simulink model "Rocket_Simulink"  (R2024b)
settings: Solver=VariableStepAuto  StartTime=0.0  StopTime=50  RelTol=1e-3
values from neighbouring files (symbols this model uses):
  A_alt = [ ... (first row only)    [linear_model.m]
  A_att = [ ... (first row only)    [linear_model.m]
  B_alt = [ ... (first row only)    [linear_model.m]
  B_att = [ ... (first row only)    [linear_model.m]
  C_alt = eye(2)    [linear_model.m]
  g = 9.82    [linear_model.m]
  h = 0.4    [linear_model.m]
  K_alt = lqr(A_alt, B_alt, Q_alt, R_alt)    [linear_model.m]
  K_att = K_aug(:, 1:6)    [linear_model.m]
  K_I = K_aug(:, 7)    [linear_model.m]
  m = 3    [linear_model.m]
undefined symbols (not defined in the file or in its folder): C_I
libraries: simulink x3, simulink_extras x1
settings Model: Creator=akewi  LastModifiedBy=akewi

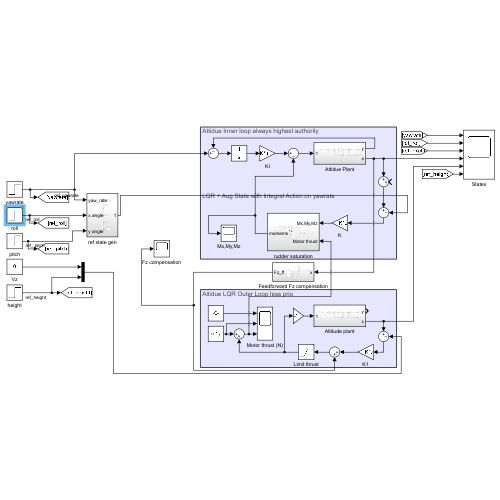
[thumbnail: Simulink's stored preview of the top-level diagram]
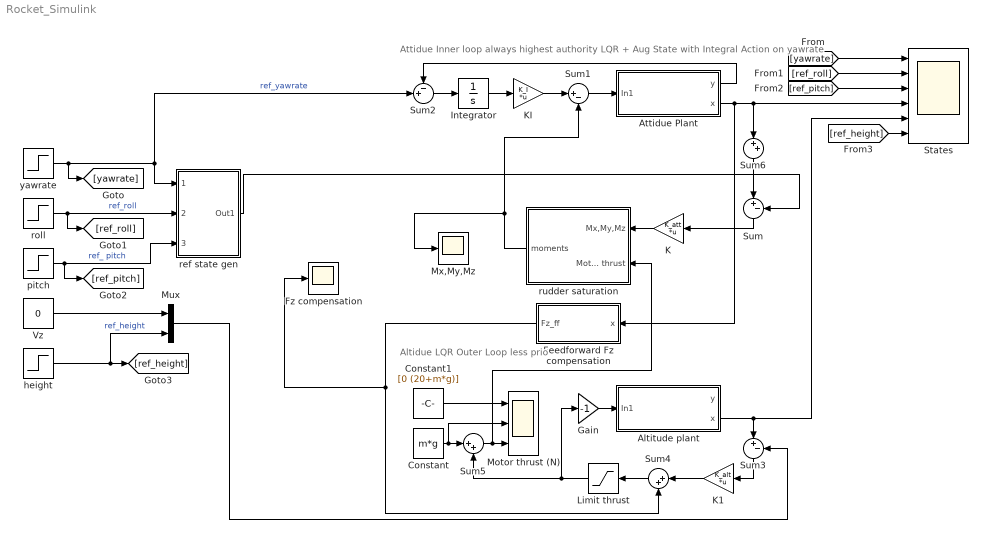
== system Rocket_Simulink ==
  note: Attidue Inner loop always highest authority
      |
      |
      |
      |
      |
      |
      |
      |
      | LQR + Aug State with Integral Action on yawrate
  note: Altidue LQR Outer Loop less prio
  Altitude plant : Subsystem
  Attidue Plant : Subsystem
  Constant : Constant  Value=m*g
  Constant1 : Constant  Value=[0 (20+m*g)]
  Feedforward Fz compensation : Subsystem
  Fz compensation : Scope
  Gain : Gain  Gain=-1
  Integrator : Integrator
  K : Gain  Gain=K_att  Multiplication=Matrix(K*u)
  K1 : Gain  Gain=K_alt  Multiplication=Matrix(K*u)
  KI : Gain  Gain=K_I  Multiplication=Matrix(K*u)
  Limit thrust : Saturate  UpperLimit=20  LowerLimit=-m*g
  Motor thrust (N) : Scope  NumInputPorts=3
  Mux : Mux  Inputs=2
  Mx,My,Mz : Scope
  States : Scope  NumInputPorts=6
  Sum : Sum  Inputs=|+-
  Sum1 : Sum  Inputs=|+-
  Sum2 : Sum  Inputs=-+|
  Sum3 : Sum  Inputs=|+-
  Sum4 : Sum  Inputs=|++
  Sum5 : Sum  Inputs=|++
  Sum6 : Sum  Inputs=|++
  Vz : Constant  Value=0
  height : Step  After=0  SampleTime=0
  pitch : Step  After=0  SampleTime=0
  ref state gen : Subsystem
  roll : Step  Time=3  After=5  SampleTime=0
  rudder saturation : Subsystem
  yawrate : Step  Time=5  After=0  SampleTime=0
  wires:
  yawrate/1 -> [yawrate], ref state gen/1(yaw_rate), Sum2/2  "ref_yawrate"
  roll/1 -> [ref_roll], ref state gen/2(x angle)  "ref_roll"
  pitch/1 -> [ref_pitch], ref state gen/3(y angle)  "ref_ pitch"
  Attidue Plant/2(x) -> Feedforward Fz compensation/1(x), States/4, Sum6/1
  ref state gen/1(Out1) -> Sum/2
  Sum/1 -> K/1
  Attidue Plant/1(y) -> Sum2/1
  Sum1/1 -> Attidue Plant/1(In1)
  KI/1 -> Sum1/1
  Integrator/1 -> KI/1
  Sum2/1 -> Integrator/1
  [yawrate] -> States/1
  [ref_roll] -> States/2
  [ref_pitch] -> States/3
  Limit thrust/1 -> Gain/1, Sum5/2
  Altitude plant/2(x) -> States/5, Sum3/1
  Sum3/1 -> K1/1
  Mux/1 -> Sum3/2
  Vz/1 -> Mux/1
  height/1 -> Mux/2, [ref_height]  "ref_height"
  Sum5/1 -> rudder saturation/2(Motor thrust), Motor thrust (N)/3
  Constant/1 -> Motor thrust (N)/2, Sum5/1
  Constant1/1 -> Motor thrust (N)/1
  Gain/1 -> Altitude plant/1(In1)
  [ref_height] -> States/6
  Sum4/1 -> Limit thrust/1
  K1/1 -> Sum4/1
  Feedforward Fz compensation/1(Fz_ff) -> Fz compensation/1, Sum4/2
  K/1 -> rudder saturation/1(Mx,My,Mz)
  rudder saturation/1(moments) -> Mx,My,Mz/1, Sum1/2
  Sum6/1 -> Sum/1

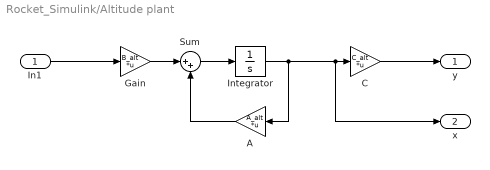
== system Rocket_Simulink/Altitude plant ==
  In1 : Inport
  A : Gain  Gain=A_alt  Multiplication=Matrix(K*u)
  C : Gain  Gain=C_alt  Multiplication=Matrix(K*u)
  Gain : Gain  Gain=B_alt  Multiplication=Matrix(K*u)
  Integrator : Integrator
  Sum : Sum  Inputs=|++
  y : Outport
  x : Outport  Port=2
  wires:
  Integrator/1 -> A/1, x/1, C/1
  C/1 -> y/1
  A/1 -> Sum/2
  Sum/1 -> Integrator/1
  Gain/1 -> Sum/1
  In1/1 -> Gain/1

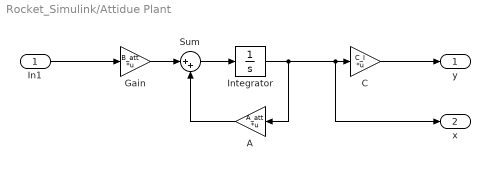
== system Rocket_Simulink/Attidue Plant ==
  In1 : Inport
  A : Gain  Gain=A_att  Multiplication=Matrix(K*u)
  C : Gain  Gain=C_I  Multiplication=Matrix(K*u)
  Gain : Gain  Gain=B_att  Multiplication=Matrix(K*u)
  Integrator : Integrator
  Sum : Sum  Inputs=|++
  y : Outport
  x : Outport  Port=2
  wires:
  Integrator/1 -> A/1, x/1, C/1
  C/1 -> y/1
  A/1 -> Sum/2
  Sum/1 -> Integrator/1
  Gain/1 -> Sum/1
  In1/1 -> Gain/1

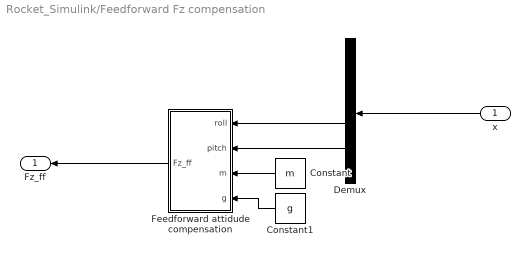
== system Rocket_Simulink/Feedforward Fz compensation ==
  x : Inport
  Constant : Constant  Value=m
  Constant1 : Constant  Value=g
  Demux : Demux  Outputs=6
  Feedforward attidude compensation : MATLAB Function  TreatAsAtomicUnit=on
  Fz_ff : Outport
  wires:
  x/1 -> Demux/1
  Feedforward attidude compensation/1(Fz_ff) -> Fz_ff/1
  Demux/4 -> Feedforward attidude compensation/1(roll)
  Demux/5 -> Feedforward attidude compensation/2(pitch)
  Constant/1 -> Feedforward attidude compensation/3(m)
  Constant1/1 -> Feedforward attidude compensation/4(g)

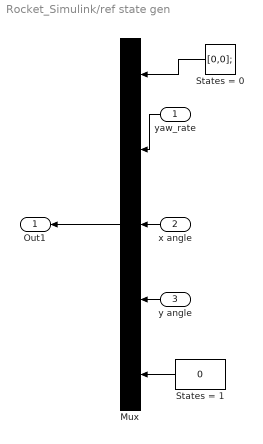
== system Rocket_Simulink/ref state gen ==
  yaw_rate : Inport
  x angle : Inport  Port=2
  y angle : Inport  Port=3
  Mux : Mux  Inputs=5
  States = 0 : Constant  Value=[0,0];
  States = 1 : Constant  Value=0
  Out1 : Outport
  wires:
  x angle/1 -> Mux/3
  States = 1/1 -> Mux/5
  y angle/1 -> Mux/4
  States = 0/1 -> Mux/1
  yaw_rate/1 -> Mux/2
  Mux/1 -> Out1/1

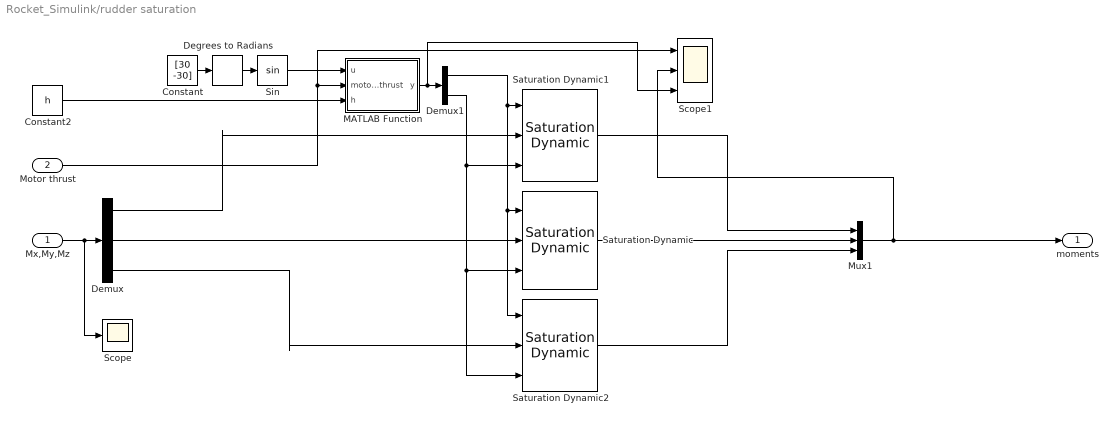
== system Rocket_Simulink/rudder saturation ==
  Mx,My,Mz : Inport
  Motor thrust : Inport  Port=2
  Constant : Constant  Value=[30 -30]
  Constant2 : Constant  Value=h
  Degrees to Radians : simulink_extras/Transformations/Degrees to Radians
  Demux : Demux  Outputs=3
  Demux1 : Demux  Outputs=2
  MATLAB Function : MATLAB Function  TreatAsAtomicUnit=on
  Mux1 : Mux  Inputs=3
  Saturation Dynamic : simulink/Discontinuities/Saturation Dynamic  OutMin=[]  OutMax=[]  OutDataTypeStr=Inherit: Same as second input  OutDataType=fixdt(1, 16)  OutScaling=2^-10  DoSatur=off
  Saturation Dynamic1 : simulink/Discontinuities/Saturation Dynamic  OutMin=[]  OutMax=[]  OutDataTypeStr=Inherit: Same as second input  OutDataType=fixdt(1, 16)  OutScaling=2^-10  DoSatur=off
  Saturation Dynamic2 : simulink/Discontinuities/Saturation Dynamic  OutMin=[]  OutMax=[]  OutDataTypeStr=Inherit: Same as second input  OutDataType=fixdt(1, 16)  OutScaling=2^-10  DoSatur=off
  Scope : Scope
  Scope1 : Scope  NumInputPorts=3
  Sin : Trigonometry
  moments : Outport
  wires:
  Mx,My,Mz/1 -> Scope/1, Demux/1
  Motor thrust/1 -> Scope1/1, MATLAB Function/2(motor_thrust)
  Demux1/2 -> Saturation Dynamic1/3, Saturation Dynamic2/3, Saturation Dynamic/3
  Mux1/1 -> Scope1/2, moments/1
  Degrees to Radians/1 -> Sin/1
  Demux1/1 -> Saturation Dynamic2/1, Saturation Dynamic/1, Saturation Dynamic1/1
  Constant/1 -> Degrees to Radians/1
  Sin/1 -> MATLAB Function/1(u)
  MATLAB Function/1(y) -> Scope1/3, Demux1/1
  Saturation Dynamic1/1 -> Mux1/1
  Saturation Dynamic/1 -> Mux1/2
  Saturation Dynamic2/1 -> Mux1/3
  Demux/1 -> Saturation Dynamic1/2
  Demux/2 -> Saturation Dynamic/2
  Demux/3 -> Saturation Dynamic2/2
  Constant2/1 -> MATLAB Function/3(h)

== matlab function Rocket_Simulink/rudder saturation/MATLAB Function ==
  data: u input; y output; motor_thrust input; h input
function y = fcn(u, motor_thrust,h)
  
y = u.*motor_thrust*h;

== matlab function Rocket_Simulink/Feedforward Fz compensation/Feedforward attidude compensation ==
  data: roll input; Fz_ff output; pitch input; m input; g input
function Fz_ff = fcn(roll,pitch,m,g)

Fz_ff = ((m*g)/(cos((roll*pi)/180)*cos((pitch*pi)/180))) -m*g;
